simulink model "Libration_model"  (R2021b)
settings: Solver=VariableStepAuto  StartTime=0.0  StopTime=tfinal  RelTol=1e-3
undefined symbols (not defined in the file or in its folder): Param
libraries: simulink_extras x1, slpidlib x1
settings Model: Creator=kmkar  LastModifiedBy=kmkar

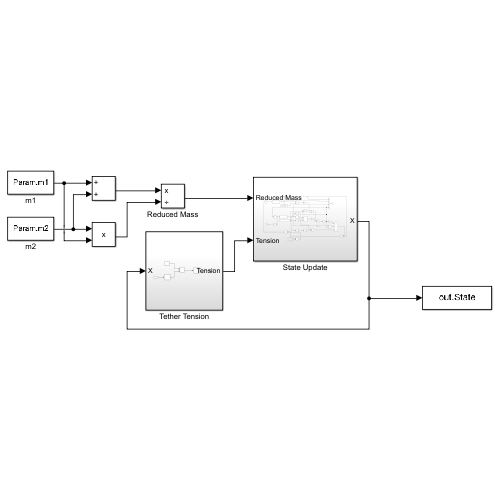
[thumbnail: Simulink's stored preview of the top-level diagram]
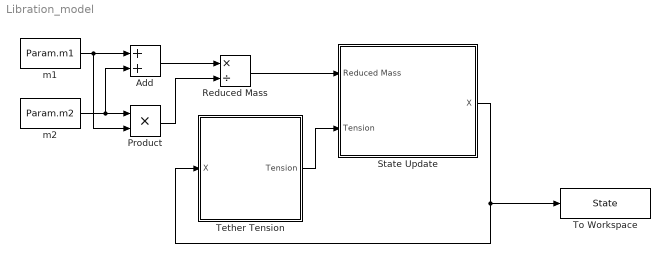
== system Libration_model ==
  Add : Sum
  Product : Product
  Reduced Mass : Product  Inputs=*/
  State Update : Subsystem
  Tether Tension : Subsystem
  To Workspace : ToWorkspace  VariableName=State  SaveFormat=Timeseries  SampleTime=-1
  m1 : Constant  Value=Param.m1
  m2 : Constant  Value=Param.m2
  wires:
  Add/1 -> Reduced Mass/1
  State Update/1(X) -> To Workspace/1, Tether Tension/1(X)
  Tether Tension/1(Tension) -> State Update/2(Tension)
  Reduced Mass/1 -> State Update/1(Reduced Mass)
  Product/1 -> Reduced Mass/2
  m2/1 -> Add/2, Product/1
  m1/1 -> Add/1, Product/2

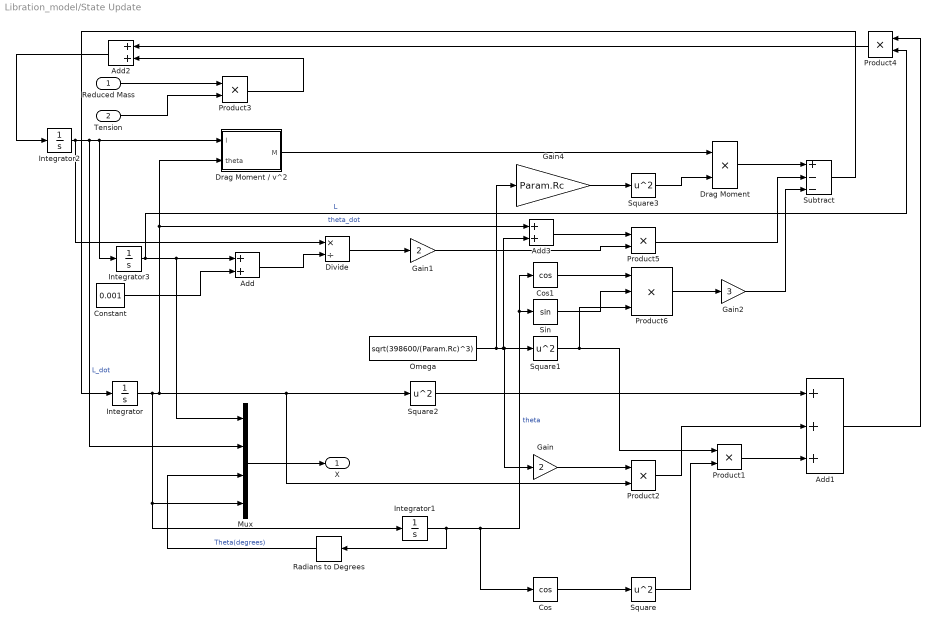
== system Libration_model/State Update ==
  Reduced Mass : Inport
  Tension : Inport  Port=2
  Add : Sum
  Add1 : Sum  Inputs=+++
  Add2 : Sum
  Add3 : Sum
  Constant : Constant  Value=0.001
  Cos : Trigonometry  Operator=cos
  Cos1 : Trigonometry  Operator=cos
  Divide : Product  Inputs=*/
  Drag Moment : Product
  Drag Moment / v^2 : MATLAB Function  TreatAsAtomicUnit=on
  Gain : Gain  Gain=2
  Gain1 : Gain  Gain=2
  Gain2 : Gain  Gain=3
  Gain4 : Gain  Gain=Param.Rc
  Integrator : Integrator
  Integrator1 : Integrator  InitialCondition=Param.theta_init
  Integrator2 : Integrator  InitialCondition=Param.Ldot_init
  Integrator3 : Integrator
  Mux : Mux
  Omega : Constant  Value=sqrt(398600/(Param.Rc)^3)
  Product{1..5} (5 alike) : Product
  Product6 : Product  Inputs=3
  Radians to Degrees : simulink_extras/Transformations/Radians to Degrees
  Sin : Trigonometry
  Square{,1..3} (4 alike) : Math  Operator=square  SaturateOnIntegerOverflow=on
  Subtract : Sum  Inputs=+--
  X : Outport
  wires:
  Constant/1 -> Add/2
  Drag Moment / v^2/1(M) -> Drag Moment/1
  Gain/1 -> Product2/1
  Product4/1 -> Add2/1
  Reduced Mass/1 -> Product3/1
  Gain1/1 -> Product5/2
  Radians to Degrees/1 -> Mux/3  "Theta(degrees)"
  Sin/1 -> Product6/2
  Gain2/1 -> Subtract/3
  Drag Moment/1 -> Subtract/1
  Integrator2/1 -> Drag Moment / v^2/1(l), Integrator3/1, Mux/2, Divide/1  "L_dot"
  Add2/1 -> Integrator2/1
  Product2/1 -> Add1/2
  Gain4/1 -> Square3/1
  Square3/1 -> Drag Moment/2
  Add/1 -> Divide/2
  Add3/1 -> Product5/1
  Cos/1 -> Square/1
  Product1/1 -> Add1/3
  Divide/1 -> Gain1/1
  Square2/1 -> Add1/1
  Tension/1 -> Product3/2
  Product5/1 -> Subtract/2
  Subtract/1 -> Integrator/1
  Add1/1 -> Product4/1
  Integrator/1 -> Integrator1/1, Mux/4, Product2/2, Square2/1, Drag Moment / v^2/2(theta), Add3/1  "theta_dot"
  Square/1 -> Product1/2
  Cos1/1 -> Product6/1
  Product3/1 -> Add2/2
  Omega/1 -> Gain/1, Square1/1, Add3/2, Gain4/1
  Product6/1 -> Gain2/1
  Mux/1 -> X/1
  Integrator1/1 -> Sin/1, Cos1/1, Cos/1, Radians to Degrees/1  "theta"
  Square1/1 -> Product1/1, Product6/3
  Integrator3/1 -> Mux/1, Add/1, Product4/2  "L"

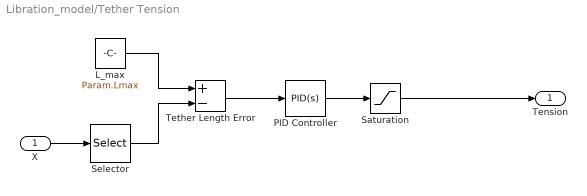
== system Libration_model/Tether Tension ==
  X : Inport
  L_max : Constant  Value=Param.Lmax
  PID Controller : slpidlib/PID Controller  Controller=PID  Form=Parallel  TimeDomain=Continuous-time  UseExternalTs=off  SampleTime=-1  IntegratorMethod=Forward Euler  FilterMethod=Forward Euler  ControllerParametersSource=internal  P=4.6  I=0  D=3.6  UseFilter=on  N=100  TunerSelectOption=Transfer Function Based (PID Tuner App)  InitialConditionSource=internal  InitialConditionForIntegrator=0  InitialConditionForFilter=0  DifferentiatorICPrevScaledInput=0  ExternalReset=none  TrackingMode=off  Kt=1  LimitOutput=off  SatLimitsSource=internal  UpperSaturationLimit=inf  LowerSaturationLimit=-inf  LinearizeAsGain=on  AntiWindupMode=none  Kb=1  POutMin=[]  POutMax=[]  IOutMin=[]  IOutMax=[]  DOutMin=[]  DOutMax=[]  NOutMin=[]  NOutMax=[]  SumOutMin=[]  SumOutMax=[]  SaturationOutMin=[]  SaturationOutMax=[]  PParamMin=[]  PParamMax=[]  IParamMin=[]  IParamMax=[]  DParamMin=[]  DParamMax=[]  NParamMin=[]  NParamMax=[]  KbParamMin=[]  KbParamMax=[]  KtParamMin=[]  KtParamMax=[]  KbOutMin=[]  KbOutMax=[]  KtOutMin=[]  KtOutMax=[]  IntegratorOutMin=[]  IntegratorOutMax=[]  FilterOutMin=[]  FilterOutMax=[]  SumI1OutMin=[]  SumI1OutMax=[]  SumI2OutMin=[]  SumI2OutMax=[]  SumI3OutMin=[]  SumI3OutMax=[]  SumI4OutMin=[]  SumI4OutMax=[]  SumDOutMin=[]  SumDOutMax=[]  DifferentiatorOutMin=[]  DifferentiatorOutMax=[]  FilterDiffOutCoefMin=[]  FilterDiffOutCoefMax=[]  ReciprocalOutMin=[]  ReciprocalOutMax=[]  SumDenOutMin=[]  SumDenOutMax=[]  SumNumOutMin=[]  SumNumOutMax=[]  DivideOutMin=[]  DivideOutMax=[]  UdiffTsProdOutMin=[]  UdiffTsProdOutMax=[]  NTsProdOutMin=[]  NTsProdOutMax=[]  UintegralTsProdOutMin=[]  UintegralTsProdOutMax=[]  UngainTsProdOutMin=[]  UngainTsProdOutMax=[]  IntegratorContinuousStateAttributes=''  IntegratorStateMustResolveToSignalObject=off  IntegratorRTWStateStorageClass=Auto  FilterContinuousStateAttributes=''  FilterStateMustResolveToSignalObject=off  FilterRTWStateStorageClass=Auto  ParallelPVariant=InternalParameters  IdealPVariant=Disabled  IVariant=InternalParameters  DVariant=InternalParameters  IntegratorVariant=Continuous  SatVariant=Disabled  AWVariant=Passthrough  PCopyVariant=Disabled  TRVariant=Disabled  FdbkBlocksVariant=Forward  IdealPFdbkVariant=Disabled  SatFdbkVariant=Disabled  DerivativeFilterVariant=ContFilter  NVariant=InternalParameters  NCopyVariant=Disabled  FilterICVariant=InternalICsFilter  IntegratorICVariant=InternalICs  ExternalResetVariant=Disabled  TRSumVariant=Passthrough  SumFdbkVariant=Disabled  SumVariant=Sum_PID  TsampFilterVariant=InternalTs  TsampNgainVariant=Passthrough  TsampIntegralVariant=Passthrough  ExternalSaturationOutDataTypeStr=Inherit: Same as second input
  Saturation : Saturate  UpperLimit=5  LowerLimit=-5
  Selector : Selector  InputPortWidth=4  IndexOptions=Index vector (dialog)  Indices=[1]  OutputSizes=1
  Tether Length Error : Sum  Inputs=+-
  Tension : Outport
  wires:
  X/1 -> Selector/1
  Selector/1 -> Tether Length Error/2
  L_max/1 -> Tether Length Error/1
  Tether Length Error/1 -> PID Controller/1
  PID Controller/1 -> Saturation/1
  Saturation/1 -> Tension/1

== matlab function Libration_model/State Update/Drag Moment // v^2 ==
  data: l input; M output; theta input
function M = fcn(l, theta)

    M = 0.5*(0.005*1.8*((1/3)^2-(1/6)^2)*l^2 - 0.022*l/3)*0.5*5.68e-13*cos(theta);
